simulink model "VectorCtrl_Asynchronous"  (Simulink 7.9)
settings: Solver=ode23tb  StartTime=0.0  StopTime=1  RelTol=1e-3
InitFcn:
  | np=2;
  | fN=50;
  | VN=400;
  | PN=3.7e+04;
  | IN=PN/(VN*1.732);
  | 
  | Rs=0.08233;
  | Lls=0.000724;
  | Rr=0.0503;
  | Llr=0.000724;
  | Lm=0.02711;
  | Ls=Lm+Lls;
  | Lr=Lm+Llr;
  | Kleak=1-Lm*Lm/(Ls*Lr);
  | Tr=Lr/Rr;
  | 
  | Ts=20e-6;
  | fbase=50;
  | Vbase=220*sqrt(3);
  | wbase=2*pi*fbase;
libraries: powerlib x11, simulink x7, powerlib_extras x6
settings Model: Creator=H002220  LastModifiedBy=H002220

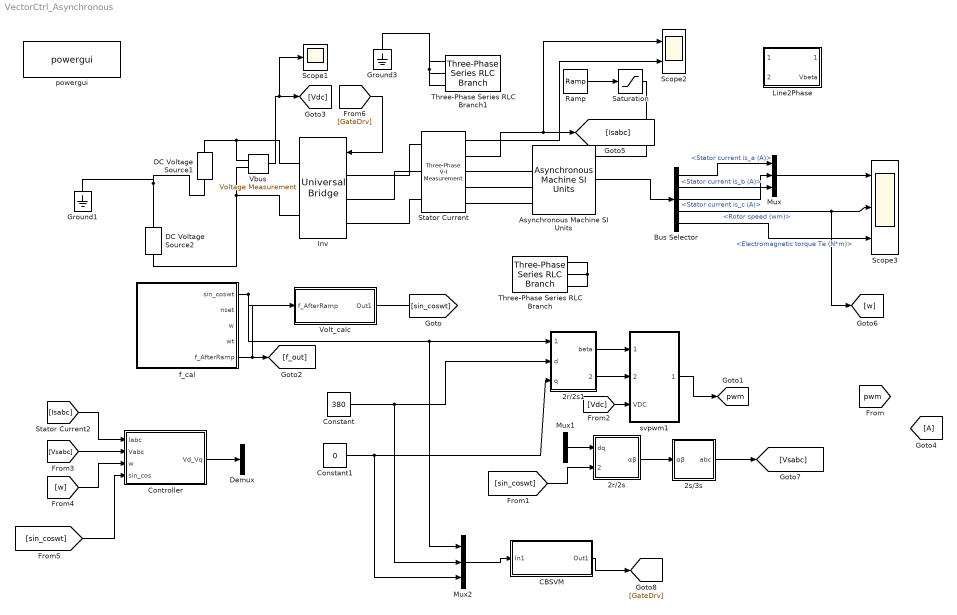
== system VectorCtrl_Asynchronous ==
  2r/2s : Subsystem
  2r/2s1 : Subsystem
  2s/3s : Subsystem
  Asynchronous Machine SI Units : powerlib/Machines/Asynchronous Machine SI Units  PresetModel="18:  50 HP (37KW)   400 V 50Hz 1480 RPM"  MechanicalLoad=Torque Tm  ShowDetailedParameters=on  RotorType=Squirrel-cage  ReferenceFrame=Rotor  NominalParameters=[3.7e+04 400 50]  Stator=[0.08233 0.000724]  Rotor=[0.0503 0.000724]  Cage1=[ 0.022 0.226/377]  Cage2=[ 0.022 0.226/377]  Lm=0.02711  Mechanical=[0.37 0.02791 2]  PolePairs=2  InitialConditions=[1 0 0 0 0 0 0 0]  Units=SI  LoadFlowParameters=1492000  SimulateSaturation=off  Saturation=[14.03593122, 27.81365428, 53.79336849, 72.68890987, 97.98006896, 148.6815601, 215.7428561, 302.9841135, 420.4778367 ; 230, 322, 414, 460, 506, 552, 598, 644, 690]  TsPowergui=0  TsBlock=-1  IterativeModel=Forward Euler  Pmec=0
  Bus Selector : BusSelector  OutputSignals=Stator measurements.Stator current is_a (A),Stator measurements.Stator current is_b (A),Stator measurements.Stator current is_c (A),Mechanical.Rotor speed (wm),Mechanical.Electromagnetic torque Te (N*m)
  CBSVM : Subsystem
  Constant : Constant  Value=380
  Constant1 : Constant  Value=0
  Controller : Subsystem
  DC Voltage Source1 : powerlib/Electrical Sources/DC Voltage Source  Amplitude=300  Measurements=None
  DC Voltage Source2 : powerlib/Electrical Sources/DC Voltage Source  Amplitude=300  Measurements=None
  Demux : Demux  Outputs=2
  Ground1 : powerlib/Elements/Ground  LConnTagsString=a
  Ground3 : powerlib/Elements/Ground  LConnTagsString=a
  Inv : powerlib/Power Electronics/Universal Bridge  Arms=3  SnubberResistance=1e5  SnubberCapacitance=inf  Device=IGBT / Diodes  Ron=1e-3  Lon=0  ForwardVoltages="[  0  0  ]"  ForwardVoltage=0  GTOparameters=[ 10e-6 , 20e-6 ]  IGBTparameters=[ 1e-6 , 2e-6 ]  Measurements=Device voltages  Measurements_2=None  converterType=Rectifier
  Line2Phase : MATLAB Function  TreatAsAtomicUnit=on
  Mux : Mux  Inputs=3
  Mux1 : Mux  Inputs=2
  Mux2 : Mux  Inputs=3
  Ramp : simulink/Sources/Ramp  slope=4  start=0  X0=0
  Saturation : Saturate  UpperLimit=20  LowerLimit=0
  Scope1 : Scope
      settings: SaveName=ScopeData3
  Scope2 : Scope  NumInputPorts=2
      settings: YMin=-5~-5  YMax=5~5  SaveName=ScopeData4
  Scope3 : Scope  NumInputPorts=3
      settings: YMin=-5~-5~-5  YMax=5~5~5  SaveName=ScopeData5
  Stator Current : powerlib/Measurements/Three-Phase V-I Measurement  VoltageMeasurement=phase-to-phase  SetLabelV=off  LabelV=Vabc  Vpu=off  VpuLL=off  CurrentMeasurement=yes  SetLabelI=off  LabelI=Iabc  Ipu=off  Pbase=100e6  Vbase=500e3  OutputType=Complex  PhasorSimulation=off  PSBequivalent=0
  Three-Phase Series RLC Branch : powerlib/Elements/Three-Phase Series RLC Branch  LConnTagsString=A|B|C  RConnTagsString=A|B|C  BranchType=RL  Resistance=1  Inductance=1e-3  Capacitance=1e-6  Measurements=None
  Three-Phase Series RLC Branch1 : powerlib/Elements/Three-Phase Series RLC Branch  LConnTagsString=A|B|C  RConnTagsString=A|B|C  BranchType=R  Resistance=1  Inductance=100*pi*Ls  Capacitance=1e-6  Measurements=None
  Vbus : powerlib/Measurements/Voltage Measurement  PhasorSimulation=off  OutputType=Complex  PSBequivalent=0
  Volt_calc : Subsystem
  f_cal : Subsystem
  powergui : powerlib/powergui  SimulationMode=Discrete  SolverType=Tustin  SampleTime=20e-6  frequency=60  SPID=off  DisableSnubberDevices=off  DisableRonSwitches=off  DisableVfSwitches=off  SwTol=0  Interpol=off  DisplayEquations=off  FunctionMessages=off  frequencyindice=0  Pbase=100e6  ErrMax=1e-4  Iterations=50  UnitsV=kV  UnitsW=MW  echomessages=off  HookPort=off  EnableUseOfTLC=off  x0status=blocks  RestoreLinks=warning  ResistiveCurrentMeasurement=off  Frange=[0:2:500]  Ylog=off  Xlog=on  ShowGrid=off  save=off  variable=ZData  structure=ScopeData4  ZoomFFT=off  StartTime=0.08  cycles=1  DisplayStyle=2  fundamental=50  FreqAxis=on  MaxFrequency=1000  frequencyindicesteady=1  RmsSteady=1  display=off  Ts=0  methode=off
  svpwm1 : Subsystem
  tag scope: pwm=global
  wires:
  2r/2s1/2(alpha) -> svpwm1/2(usaref)
  2r/2s1/1(beta) -> svpwm1/1(usbref)
  [Vdc] -> svpwm1/3(VDC)
  Vbus/1 -> [Vdc], Scope1/1
  Stator Current/2 -> [Isabc], Scope2/1
  f_cal/5(f_AfterRamp) -> [f_out], Volt_calc/1(f_AfterRamp)
  f_cal/1(sin_coswt) -> [sin_coswt], 2r/2s1/1(sin_cos), Mux2/1
  Asynchronous Machine SI Units/1 -> Bus Selector/1
  Ramp/1 -> Saturation/1
  Saturation/1 -> Asynchronous Machine SI Units/1
  Bus Selector/1 -> Mux/1  "<Stator current is_a (A)>"
  Bus Selector/2 -> Mux/2  "<Stator current is_b (A)>"
  Bus Selector/3 -> Mux/3  "<Stator current is_c (A)>"
  Mux/1 -> Scope3/1
  Bus Selector/4 -> Scope3/2, [w]  "<Rotor speed (wm)>"
  Bus Selector/5 -> Scope3/3  "<Electromagnetic torque Te (N*m)>"
  [Isabc] -> Controller/1(Iabc)
  [Vsabc] -> Controller/2(Vabc)
  [w] -> Controller/3(w)
  Mux1/1 -> 2r/2s/1(dq)
  [sin_coswt] -> 2r/2s/2(sin_cos)
  2r/2s/1(αβ) -> 2s/3s/1(αβ)
  2s/3s/1(abc) -> [Vsabc]
  [sin_coswt] -> Controller/4(sin_cos)
  Controller/1(Vd_Vq) -> Demux/1
  Constant/1 -> 2r/2s1/2(d), Mux2/2
  Constant1/1 -> 2r/2s1/3(q), Mux2/3
  Mux2/1 -> CBSVM/1(In1)
  Stator Current/1 -> Scope2/2
  svpwm1/1(6pulse) -> [pwm]
  CBSVM/1(Out1) -> [GateDrv]
  [GateDrv] -> Inv/1
  connections:
  Inv/LConn1 -- Stator Current/LConn1
  Inv/LConn2 -- Stator Current/LConn2
  Inv/LConn3 -- Stator Current/LConn3
  Inv/RConn2 -- Vbus/LConn2 -- DC Voltage Source2/LConn1
  DC Voltage Source1/RConn1 -- Inv/RConn1 -- Vbus/LConn1
  Ground3/LConn1 -- Three-Phase Series RLC Branch1/LConn1 -- Three-Phase Series RLC Branch1/LConn3 -- Three-Phase Series RLC Branch1/LConn2
  DC Voltage Source2/RConn1 -- DC Voltage Source1/LConn1 -- Ground1/LConn1
  Three-Phase Series RLC Branch/RConn1 -- Three-Phase Series RLC Branch/RConn3 -- Three-Phase Series RLC Branch/RConn2
  Stator Current/RConn1 -- Asynchronous Machine SI Units/LConn1
  Stator Current/RConn2 -- Asynchronous Machine SI Units/LConn2
  Stator Current/RConn3 -- Asynchronous Machine SI Units/LConn3

== system VectorCtrl_Asynchronous/2r/2s ==
  dq : Inport
  sin_cos : Inport  Port=2
  Demux : Demux  Outputs=2
  Demux1 : Demux  Outputs=2
  MATLAB Function : MATLAB Function  TreatAsAtomicUnit=on
  Mux : Mux  Inputs=2
  αβ : Outport
  wires:
  Mux/1 -> αβ/1
  Demux/2 -> MATLAB Function/4(coswt)
  Demux/1 -> MATLAB Function/3(sinwt)
  sin_cos/1 -> Demux/1
  dq/1 -> Demux1/1
  Demux1/1 -> MATLAB Function/1(Vd)
  Demux1/2 -> MATLAB Function/2(Vq)
  MATLAB Function/1(Valpha) -> Mux/1
  MATLAB Function/2(Vbeta) -> Mux/2

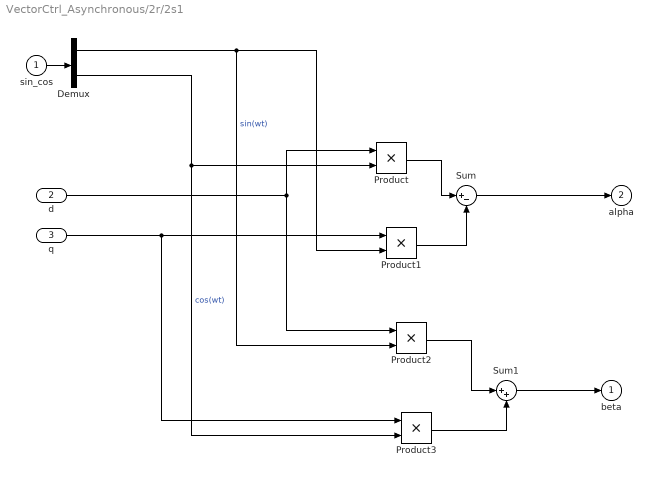
== system VectorCtrl_Asynchronous/2r/2s1 ==
  sin_cos : Inport  PortDimensions=2
  d : Inport  Port=2
  q : Inport  Port=3
  Demux : Demux  Outputs=2
  Product{,1..3} (4 alike) : Product  RndMeth=Zero
  Sum : Sum  Inputs=|+-
  Sum1 : Sum  Inputs=|++
  beta : Outport  InitialOutput=0
  alpha : Outport  Port=2  InitialOutput=0
  wires:
  Sum/1 -> alpha/1
  Demux/1 -> Product1/2, Product2/2  "sin(wt)"
  Demux/2 -> Product/2, Product3/2  "cos(wt)"
  sin_cos/1 -> Demux/1
  d/1 -> Product/1, Product2/1
  q/1 -> Product1/1, Product3/1
  Product/1 -> Sum/1
  Product1/1 -> Sum/2
  Product2/1 -> Sum1/1
  Product3/1 -> Sum1/2
  Sum1/1 -> beta/1

== system VectorCtrl_Asynchronous/2s/3s ==
  αβ : Inport
  Demux : Demux  Outputs=2
  MATLAB Function : MATLAB Function  TreatAsAtomicUnit=on
  Mux : Mux  Inputs=3
  abc : Outport
  wires:
  Demux/1 -> MATLAB Function/1(Valpha)
  Demux/2 -> MATLAB Function/2(Vbeta)
  MATLAB Function/1(Va) -> Mux/1
  MATLAB Function/2(Vb) -> Mux/2
  MATLAB Function/3(Vc) -> Mux/3
  Mux/1 -> abc/1
  αβ/1 -> Demux/1

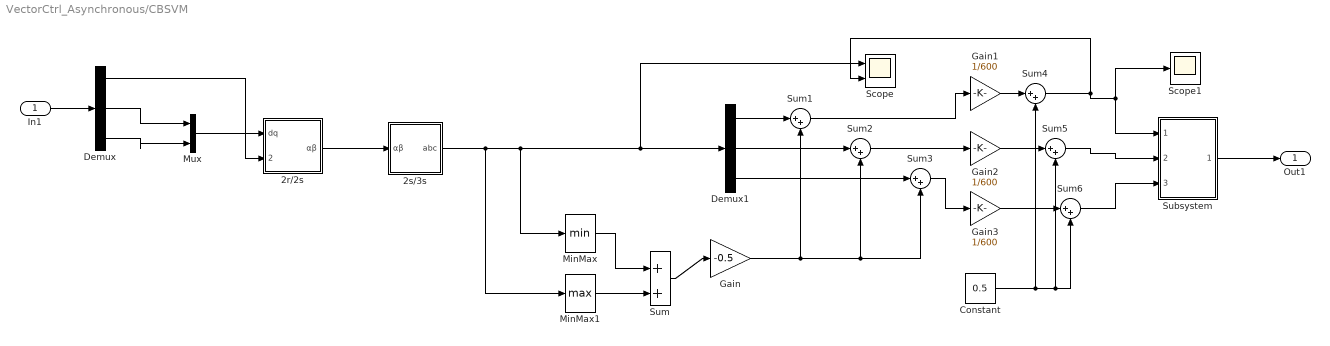
== system VectorCtrl_Asynchronous/CBSVM ==
  In1 : Inport
  2r/2s : Subsystem
  2s/3s : Subsystem
  Constant : Constant  Value=0.5
  Demux : Demux  Outputs=3
  Demux1 : Demux  Outputs=3
  Gain : Gain  Gain=-0.5
  Gain1 : Gain  Gain=1/600
  Gain2 : Gain  Gain=1/600
  Gain3 : Gain  Gain=1/600
  MinMax : MinMax
  MinMax1 : MinMax  Function=max
  Mux : Mux  Inputs=2
  Scope : Scope  NumInputPorts=2
      settings: YMin=-5~-5  YMax=5~5  SaveName=ScopeData12
  Scope1 : Scope
      settings: SaveName=ScopeData14
  Subsystem : Subsystem
  Sum{,1..6} (7 alike) : Sum  Inputs=|++
  Out1 : Outport
  wires:
  In1/1 -> Demux/1
  Demux/2 -> Mux/1
  Demux/3 -> Mux/2
  Mux/1 -> 2r/2s/1(dq)
  Demux/1 -> 2r/2s/2(sin_cos)
  2r/2s/1(αβ) -> 2s/3s/1(αβ)
  2s/3s/1(abc) -> MinMax/1, Demux1/1, Scope/1, MinMax1/1
  MinMax/1 -> Sum/1
  MinMax1/1 -> Sum/2
  Sum/1 -> Gain/1
  Demux1/1 -> Sum1/1
  Demux1/2 -> Sum2/1
  Demux1/3 -> Sum3/1
  Gain/1 -> Sum3/2, Sum2/2, Sum1/2
  Subsystem/1(Out1) -> Out1/1
  Sum1/1 -> Gain1/1
  Sum2/1 -> Gain2/1
  Sum3/1 -> Gain3/1
  Sum4/1 -> Subsystem/1(TCM1), Scope1/1, Scope/2
  Sum5/1 -> Subsystem/2(TCM2)
  Sum6/1 -> Subsystem/3(TCM3)
  Gain1/1 -> Sum4/1
  Gain2/1 -> Sum5/1
  Gain3/1 -> Sum6/1
  Constant/1 -> Sum6/2, Sum5/2, Sum4/2

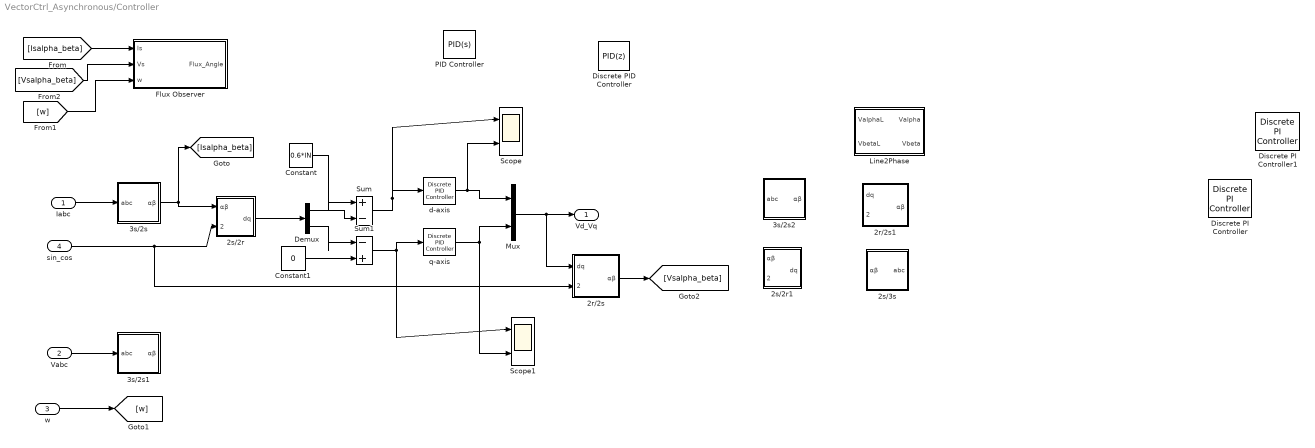
== system VectorCtrl_Asynchronous/Controller ==
  Iabc : Inport
  Vabc : Inport  Port=2
  w : Inport  Port=3
  sin_cos : Inport  Port=4
  2r/2s : Subsystem
  2r/2s1 : Subsystem
  2s/2r : Subsystem
  2s/2r1 : Subsystem
  2s/3s : Subsystem
  3s/2s : Subsystem
  3s/2s1 : Subsystem
  3s/2s2 : Subsystem
  Constant : Constant  Value=0.6*IN
  Constant1 : Constant  Value=0
  Demux : Demux  Outputs=2
  Discrete PI Controller : powerlib_extras/Discrete  Control Blocks/Discrete PI Controller  Kp=0.1  Ki=1  Par_Limits=[1e6 -1e6]  Init=0  Ts=50e-6
  Discrete PI Controller1 : powerlib_extras/Discrete  Control Blocks/Discrete PI Controller  Kp=0.1  Ki=1  Par_Limits=[1e6 -1e6]  Init=0  Ts=50e-6
  Discrete PID Controller : simulink/Continuous/PID Controller  Controller=PID  TimeDomain=Discrete-time  SampleTime=1  IntegratorMethod=Forward Euler  FilterMethod=Forward Euler  Form=Parallel  P=1  I=1  D=0  N=100  InitialConditionSource=internal  InitialConditionForIntegrator=0  InitialConditionForFilter=0  ExternalReset=none  LimitOutput=off  UpperSaturationLimit=inf  LowerSaturationLimit=-inf  LinearizeAsGain=off  AntiWindupMode=none  Kb=1  TrackingMode=off  Kt=1  PParamMin=[]  PParamMax=[]  IParamMin=[]  IParamMax=[]  DParamMin=[]  DParamMax=[]  NParamMin=[]  NParamMax=[]  KbParamMin=[]  KbParamMax=[]  KtParamMin=[]  KtParamMax=[]  POutMin=[]  POutMax=[]  IOutMin=[]  IOutMax=[]  DOutMin=[]  DOutMax=[]  NOutMin=[]  NOutMax=[]  KbOutMin=[]  KbOutMax=[]  KtOutMin=[]  KtOutMax=[]  IntegratorOutMin=[]  IntegratorOutMax=[]  FilterOutMin=[]  FilterOutMax=[]  SumOutMin=[]  SumOutMax=[]  SumI1OutMin=[]  SumI1OutMax=[]  SumI2OutMin=[]  SumI2OutMax=[]  SumI3OutMin=[]  SumI3OutMax=[]  SumDOutMin=[]  SumDOutMax=[]  SaturationOutMin=[]  SaturationOutMax=[]  IntegratorContinuousStateAttributes=''  IntegratorStateMustResolveToSignalObject=off  IntegratorRTWStateStorageClass=Auto  FilterContinuousStateAttributes=''  FilterStateMustResolveToSignalObject=off  FilterRTWStateStorageClass=Auto
  Flux Observer : Subsystem
  Line2Phase : MATLAB Function  TreatAsAtomicUnit=on
  Mux : Mux  Inputs=2
  PID Controller : simulink/Continuous/PID Controller  Controller=PID  TimeDomain=Continuous-time  SampleTime=1  IntegratorMethod=Forward Euler  FilterMethod=Forward Euler  Form=Parallel  P=1  I=1  D=0  N=100  InitialConditionSource=internal  InitialConditionForIntegrator=0  InitialConditionForFilter=0  ExternalReset=none  LimitOutput=off  UpperSaturationLimit=inf  LowerSaturationLimit=-inf  LinearizeAsGain=off  AntiWindupMode=none  Kb=1  TrackingMode=off  Kt=1  PParamMin=[]  PParamMax=[]  IParamMin=[]  IParamMax=[]  DParamMin=[]  DParamMax=[]  NParamMin=[]  NParamMax=[]  KbParamMin=[]  KbParamMax=[]  KtParamMin=[]  KtParamMax=[]  POutMin=[]  POutMax=[]  IOutMin=[]  IOutMax=[]  DOutMin=[]  DOutMax=[]  NOutMin=[]  NOutMax=[]  KbOutMin=[]  KbOutMax=[]  KtOutMin=[]  KtOutMax=[]  IntegratorOutMin=[]  IntegratorOutMax=[]  FilterOutMin=[]  FilterOutMax=[]  SumOutMin=[]  SumOutMax=[]  SumI1OutMin=[]  SumI1OutMax=[]  SumI2OutMin=[]  SumI2OutMax=[]  SumI3OutMin=[]  SumI3OutMax=[]  SumDOutMin=[]  SumDOutMax=[]  SaturationOutMin=[]  SaturationOutMax=[]  IntegratorContinuousStateAttributes=''  IntegratorStateMustResolveToSignalObject=off  IntegratorRTWStateStorageClass=Auto  FilterContinuousStateAttributes=''  FilterStateMustResolveToSignalObject=off  FilterRTWStateStorageClass=Auto
  Scope : Scope  NumInputPorts=2
      settings: YMin=-5~-5  YMax=5~5  SaveName=ScopeData7
  Scope1 : Scope  NumInputPorts=2
      settings: YMin=-5~-5  YMax=5~5  SaveName=ScopeData11
  Sum : Sum  Inputs=|+-
  Sum1 : Sum  Inputs=|-+
  d-axis : powerlib_extras/Discrete  Control Blocks/Discrete PID Controller  Kp=100  Ki=2  Kd=0  TcD=Ts/2  Par_Limits=[600 -600]  Init=0  Ts=Ts/2
  q-axis : powerlib_extras/Discrete  Control Blocks/Discrete PID Controller  Kp=100  Ki=2  Kd=0  TcD=Ts/2  Par_Limits=[600 -600]  Init=0  Ts=Ts/2
  Vd_Vq : Outport
  wires:
  Iabc/1 -> 3s/2s/1(abc)
  3s/2s/1(αβ) -> [Isalpha_beta], 2s/2r/1(αβ)
  [Isalpha_beta] -> Flux Observer/1(Is)
  w/1 -> [w]
  [w] -> Flux Observer/3(w)
  Vabc/1 -> 3s/2s1/1(abc)
  [Vsalpha_beta] -> Flux Observer/2(Vs)
  sin_cos/1 -> 2s/2r/2(sin_cos), 2r/2s/2(sin_cos)
  2s/2r/1(dq) -> Demux/1
  Demux/1 -> Sum/2
  Demux/2 -> Sum1/1
  Constant/1 -> Sum/1
  Constant1/1 -> Sum1/2
  Sum1/1 -> q-axis/1, Scope1/1
  Sum/1 -> d-axis/1, Scope/1
  d-axis/1 -> Mux/1, Scope/2
  q-axis/1 -> Mux/2, Scope1/2
  Mux/1 -> Vd_Vq/1, 2r/2s/1(dq)
  2r/2s/1(αβ) -> [Vsalpha_beta]

== system VectorCtrl_Asynchronous/Volt_calc ==
  f_AfterRamp : Inport
  Constant : Constant  Value=0.1*fbase
  Gain : Gain  Gain=1/fbase
  Gain1 : Gain  Gain=Vbase
  Ramp : simulink/Sources/Ramp  slope=1  start=0  X0=0
  Scope : Scope
      settings: SaveName=ScopeData6
  Switch : Switch
  Out1 : Outport
  wires:
  Gain/1 -> Gain1/1
  Gain1/1 -> Out1/1, Scope/1
  Ramp/1 -> Switch/2
  f_AfterRamp/1 -> Switch/1
  Constant/1 -> Switch/3
  Switch/1 -> Gain/1

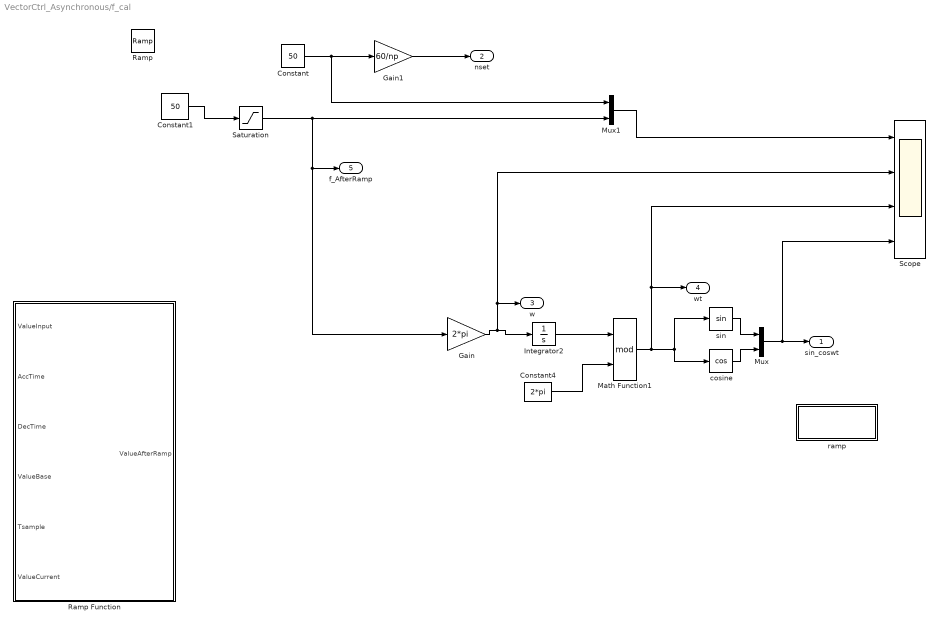
== system VectorCtrl_Asynchronous/f_cal ==
  Constant : Constant  Value=50
  Constant1 : Constant  Value=50
  Constant4 : Constant  Value=2*pi
  Gain : Gain  Gain=2*pi
  Gain1 : Gain  Gain=60/np
  Integrator2 : Integrator
  Math Function1 : Math  Operator=mod  SaturateOnIntegerOverflow=on
  Mux : Mux  Inputs=2
  Mux1 : Mux  Inputs=2
  Ramp : simulink/Sources/Ramp  slope=10  start=0  X0=0
  Ramp Function : MATLAB Function  TreatAsAtomicUnit=on
  Saturation : Saturate  UpperLimit=50  LowerLimit=0
  Scope : Scope  NumInputPorts=4
      settings: YMin=-5~-5~-5~-5  YMax=5~5~5~5
  cosine : Trigonometry  Operator=cos
  ramp : Subsystem
  sin : Trigonometry
  sin_coswt : Outport
  nset : Outport  Port=2
  w : Outport  Port=3
  wt : Outport  Port=4
  f_AfterRamp : Outport  Port=5
  wires:
  sin/1 -> Mux/1
  cosine/1 -> Mux/2
  Mux/1 -> sin_coswt/1, Scope/4
  Gain1/1 -> nset/1
  Mux1/1 -> Scope/1
  Constant4/1 -> Math Function1/2
  Integrator2/1 -> Math Function1/1
  Gain/1 -> Integrator2/1, w/1, Scope/2
  Math Function1/1 -> sin/1, cosine/1, wt/1, Scope/3
  Constant/1 -> Gain1/1, Mux1/1
  Saturation/1 -> Mux1/2, f_AfterRamp/1, Gain/1
  Constant1/1 -> Saturation/1

== system VectorCtrl_Asynchronous/svpwm1 ==
  usbref : Inport
  usaref : Inport  Port=2
  VDC : Inport  Port=3
  Campare Time Calculate : Subsystem
  Memory : Memory
  On/Off Delay : powerlib_extras/Control  Blocks/On//Off Delay  type_delay=On delay  delay=1e-6  ic=0
  Sector Calculate : Subsystem
  Subsystem : Subsystem
  T : Constant  Value=1/5000
  T1,T2 Calculate : Subsystem
  x,y,z Calculate : Subsystem
  6pulse : Outport
  wires:
  usbref/1 -> Sector Calculate/1(usbref), x,y,z Calculate/1(usbref)
  usaref/1 -> Sector Calculate/2(usaref), x,y,z Calculate/2(usaref)
  Sector Calculate/1(N) -> T1,T2 Calculate/1(N), Campare Time Calculate/1(N)
  x,y,z Calculate/1(x) -> T1,T2 Calculate/2(x)
  x,y,z Calculate/2(y) -> T1,T2 Calculate/3(y)
  x,y,z Calculate/3(z) -> T1,T2 Calculate/4(z)
  T1,T2 Calculate/1(T1) -> Campare Time Calculate/2(T1)
  T1,T2 Calculate/2(T2) -> Campare Time Calculate/3(T2)
  Campare Time Calculate/1(TCM1) -> Subsystem/1(TCM1)
  Campare Time Calculate/2(TCM2) -> Subsystem/2(TCM2)
  Campare Time Calculate/3(TCM3) -> Subsystem/3(TCM3)
  Subsystem/1(Out1) -> Memory/1
  T/1 -> x,y,z Calculate/3(T), T1,T2 Calculate/5(T), Campare Time Calculate/4(T)
  VDC/1 -> x,y,z Calculate/4(VDC)
  Memory/1 -> On/Off Delay/1
  On/Off Delay/1 -> 6pulse/1

== system VectorCtrl_Asynchronous/CBSVM/2r/2s ==
  dq : Inport
  sin_cos : Inport  Port=2
  Demux : Demux  Outputs=2
  Demux1 : Demux  Outputs=2
  MATLAB Function : MATLAB Function  TreatAsAtomicUnit=on
  Mux : Mux  Inputs=2
  αβ : Outport
  wires:
  Mux/1 -> αβ/1
  Demux/2 -> MATLAB Function/4(coswt)
  Demux/1 -> MATLAB Function/3(sinwt)
  sin_cos/1 -> Demux/1
  dq/1 -> Demux1/1
  Demux1/1 -> MATLAB Function/1(Vd)
  Demux1/2 -> MATLAB Function/2(Vq)
  MATLAB Function/1(Valpha) -> Mux/1
  MATLAB Function/2(Vbeta) -> Mux/2

== system VectorCtrl_Asynchronous/CBSVM/2s/3s ==
  αβ : Inport
  Demux : Demux  Outputs=2
  MATLAB Function : MATLAB Function  TreatAsAtomicUnit=on
  Mux : Mux  Inputs=3
  abc : Outport
  wires:
  Demux/1 -> MATLAB Function/1(Valpha)
  Demux/2 -> MATLAB Function/2(Vbeta)
  MATLAB Function/1(Va) -> Mux/1
  MATLAB Function/2(Vb) -> Mux/2
  MATLAB Function/3(Vc) -> Mux/3
  Mux/1 -> abc/1
  αβ/1 -> Demux/1

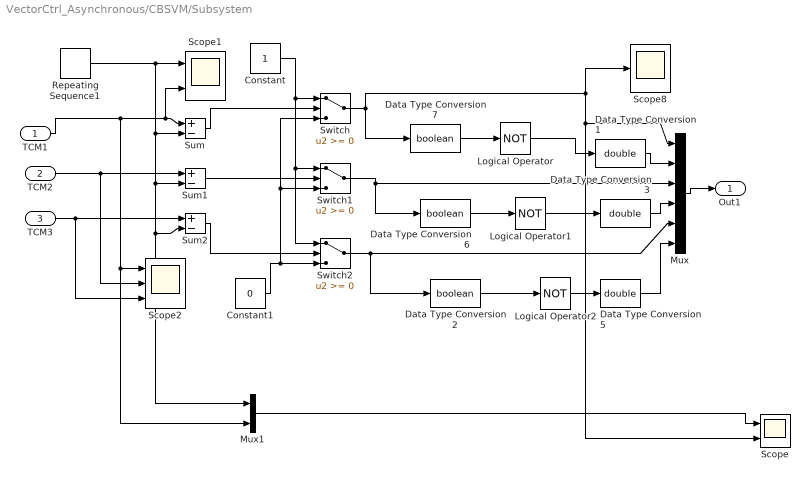
== system VectorCtrl_Asynchronous/CBSVM/Subsystem ==
  TCM1 : Inport
  TCM2 : Inport  Port=2
  TCM3 : Inport  Port=3
  Constant : Constant
  Constant1 : Constant  Value=0
  Data Type Conversion1 : DataTypeConversion  OutDataTypeStr=double  SaturateOnIntegerOverflow=on  RndMeth=Zero
  Data Type Conversion2 : DataTypeConversion  OutDataTypeStr=boolean  SaturateOnIntegerOverflow=on  RndMeth=Zero
  Data Type Conversion3 : DataTypeConversion  OutDataTypeStr=double  SaturateOnIntegerOverflow=on  RndMeth=Zero
  Data Type Conversion5 : DataTypeConversion  OutDataTypeStr=double  SaturateOnIntegerOverflow=on  RndMeth=Zero
  Data Type Conversion6 : DataTypeConversion  OutDataTypeStr=boolean  SaturateOnIntegerOverflow=on  RndMeth=Zero
  Data Type Conversion7 : DataTypeConversion  OutDataTypeStr=boolean  SaturateOnIntegerOverflow=on  RndMeth=Zero
  Logical Operator : Logic  Operator=NOT  AllPortsSameDT=off
  Logical Operator1 : Logic  Operator=NOT  AllPortsSameDT=off
  Logical Operator2 : Logic  Operator=NOT  AllPortsSameDT=off
  Mux : Mux  Inputs=6
  Mux1 : Mux  Inputs=2
  Repeating Sequence1 : simulink/Sources/Repeating Sequence  rep_seq_t=[0 1/10000 1/5000]  rep_seq_y=[0 1 0]
  Scope : Scope  NumInputPorts=2
      settings: YMin=-5~-5  YMax=5~5  SaveName=ScopeData21
  Scope1 : Scope  NumInputPorts=2
      settings: TimeRange=0.028  YMin=0~2.45e-005  YMax=1.2~2.64e-005  SaveName=ScopeData15
  Scope2 : Scope  NumInputPorts=3
      settings: TimeRange=1  YMin=2.25e-005~2.25e-005~2.25e-05  YMax=6e-005~6e-005~6e-05  SaveName=ScopeData19
  Scope8 : Scope
      settings: TimeRange=0.07000000000000001  YMin=0  YMax=2  SaveName=ScopeData13
  Sum : Sum  Inputs=+-  SaturateOnIntegerOverflow=on
  Sum1 : Sum  Inputs=+-  SaturateOnIntegerOverflow=on
  Sum2 : Sum  Inputs=+-  SaturateOnIntegerOverflow=on
  Switch : Switch  SaturateOnIntegerOverflow=on
  Switch1 : Switch  SaturateOnIntegerOverflow=on
  Switch2 : Switch  SaturateOnIntegerOverflow=on
  Out1 : Outport
  wires:
  Constant/1 -> Switch/1, Switch1/1, Switch2/1
  Constant1/1 -> Switch2/3, Switch/3, Switch1/3
  Repeating Sequence1/1 -> Scope1/1, Sum/2, Sum1/2, Sum2/2, Mux1/1
  TCM1/1 -> Sum/1, Scope1/2, Scope2/1, Mux1/2
  TCM2/1 -> Sum1/1, Scope2/2
  TCM3/1 -> Sum2/1, Scope2/3
  Sum/1 -> Switch/2
  Sum1/1 -> Switch1/2
  Sum2/1 -> Switch2/2
  Mux/1 -> Out1/1
  Switch/1 -> Scope8/1, Mux/1, Scope/2, Data Type Conversion7/1
  Switch1/1 -> Mux/3, Data Type Conversion6/1
  Switch2/1 -> Data Type Conversion2/1, Mux/5
  Logical Operator2/1 -> Data Type Conversion5/1
  Logical Operator1/1 -> Data Type Conversion3/1
  Logical Operator/1 -> Data Type Conversion1/1
  Data Type Conversion1/1 -> Mux/2
  Data Type Conversion3/1 -> Mux/4
  Data Type Conversion5/1 -> Mux/6
  Data Type Conversion7/1 -> Logical Operator/1
  Data Type Conversion6/1 -> Logical Operator1/1
  Data Type Conversion2/1 -> Logical Operator2/1
  Mux1/1 -> Scope/1

== system VectorCtrl_Asynchronous/Controller/2r/2s ==
  dq : Inport
  sin_cos : Inport  Port=2
  Demux : Demux  Outputs=2
  Demux1 : Demux  Outputs=2
  MATLAB Function : MATLAB Function  TreatAsAtomicUnit=on
  Mux : Mux  Inputs=2
  αβ : Outport
  wires:
  Mux/1 -> αβ/1
  Demux/2 -> MATLAB Function/4(coswt)
  Demux/1 -> MATLAB Function/3(sinwt)
  sin_cos/1 -> Demux/1
  dq/1 -> Demux1/1
  Demux1/1 -> MATLAB Function/1(Vd)
  Demux1/2 -> MATLAB Function/2(Vq)
  MATLAB Function/1(Valpha) -> Mux/1
  MATLAB Function/2(Vbeta) -> Mux/2

== system VectorCtrl_Asynchronous/Controller/2r/2s1 ==
  dq : Inport
  sin_cos : Inport  Port=2
  Demux : Demux  Outputs=2
  Demux1 : Demux  Outputs=2
  MATLAB Function : MATLAB Function  TreatAsAtomicUnit=on
  Mux : Mux  Inputs=2
  αβ : Outport
  wires:
  MATLAB Function/2(Vbeta) -> Mux/2
  MATLAB Function/1(Valpha) -> Mux/1
  Demux1/2 -> MATLAB Function/2(Vq)
  Demux1/1 -> MATLAB Function/1(Vd)
  dq/1 -> Demux1/1
  sin_cos/1 -> Demux/1
  Demux/1 -> MATLAB Function/3(sinwt)
  Demux/2 -> MATLAB Function/4(coswt)
  Mux/1 -> αβ/1

== system VectorCtrl_Asynchronous/Controller/2s/2r ==
  αβ : Inport
  sin_cos : Inport  Port=2
  Demux : Demux  Outputs=2
  Demux1 : Demux  Outputs=2
  MATLAB Function : MATLAB Function  TreatAsAtomicUnit=on
  Mux : Mux  Inputs=2
  dq : Outport
  wires:
  αβ/1 -> Demux1/1
  sin_cos/1 -> Demux/1
  Demux/1 -> MATLAB Function/3(sinwt)
  Demux/2 -> MATLAB Function/4(coswt)
  MATLAB Function/1(Vd) -> Mux/1
  MATLAB Function/2(Vq) -> Mux/2
  Mux/1 -> dq/1
  Demux1/2 -> MATLAB Function/2(Vbeta)
  Demux1/1 -> MATLAB Function/1(Valpha)

== system VectorCtrl_Asynchronous/Controller/2s/2r1 ==
  αβ : Inport
  sin_cos : Inport  Port=2
  Demux : Demux  Outputs=2
  Demux1 : Demux  Outputs=2
  MATLAB Function : MATLAB Function  TreatAsAtomicUnit=on
  Mux : Mux  Inputs=2
  dq : Outport
  wires:
  Demux1/1 -> MATLAB Function/1(Valpha)
  Demux1/2 -> MATLAB Function/2(Vbeta)
  Mux/1 -> dq/1
  MATLAB Function/2(Vq) -> Mux/2
  MATLAB Function/1(Vd) -> Mux/1
  Demux/2 -> MATLAB Function/4(coswt)
  Demux/1 -> MATLAB Function/3(sinwt)
  sin_cos/1 -> Demux/1
  αβ/1 -> Demux1/1

== system VectorCtrl_Asynchronous/Controller/2s/3s ==
  αβ : Inport
  Demux : Demux  Outputs=2
  MATLAB Function : MATLAB Function  TreatAsAtomicUnit=on
  Mux : Mux  Inputs=3
  abc : Outport
  wires:
  Demux/1 -> MATLAB Function/1(Valpha)
  Demux/2 -> MATLAB Function/2(Vbeta)
  MATLAB Function/1(Va) -> Mux/1
  MATLAB Function/2(Vb) -> Mux/2
  MATLAB Function/3(Vc) -> Mux/3
  Mux/1 -> abc/1
  αβ/1 -> Demux/1

== system VectorCtrl_Asynchronous/Controller/3s/2s ==
  abc : Inport
  Demux : Demux  Outputs=3
  MATLAB Function : MATLAB Function  TreatAsAtomicUnit=on
  Mux : Mux  Inputs=2
  αβ : Outport
  wires:
  abc/1 -> Demux/1
  Mux/1 -> αβ/1
  Demux/1 -> MATLAB Function/1(Va)
  Demux/2 -> MATLAB Function/2(Vb)
  Demux/3 -> MATLAB Function/3(Vc)
  MATLAB Function/1(Valpha) -> Mux/1
  MATLAB Function/2(Vbeta) -> Mux/2

== system VectorCtrl_Asynchronous/Controller/3s/2s1 ==
  abc : Inport
  Demux : Demux  Outputs=3
  MATLAB Function : MATLAB Function  TreatAsAtomicUnit=on
  Mux : Mux  Inputs=2
  αβ : Outport
  wires:
  MATLAB Function/2(Vbeta) -> Mux/2
  MATLAB Function/1(Valpha) -> Mux/1
  Demux/3 -> MATLAB Function/3(Vc)
  Demux/2 -> MATLAB Function/2(Vb)
  Demux/1 -> MATLAB Function/1(Va)
  Mux/1 -> αβ/1
  abc/1 -> Demux/1

== system VectorCtrl_Asynchronous/Controller/3s/2s2 ==
  abc : Inport
  Demux : Demux  Outputs=3
  MATLAB Function : MATLAB Function  TreatAsAtomicUnit=on
  Mux : Mux  Inputs=2
  αβ : Outport
  wires:
  abc/1 -> Demux/1
  Mux/1 -> αβ/1
  Demux/1 -> MATLAB Function/1(Va)
  Demux/2 -> MATLAB Function/2(Vb)
  Demux/3 -> MATLAB Function/3(Vc)
  MATLAB Function/1(Valpha) -> Mux/1
  MATLAB Function/2(Vbeta) -> Mux/2

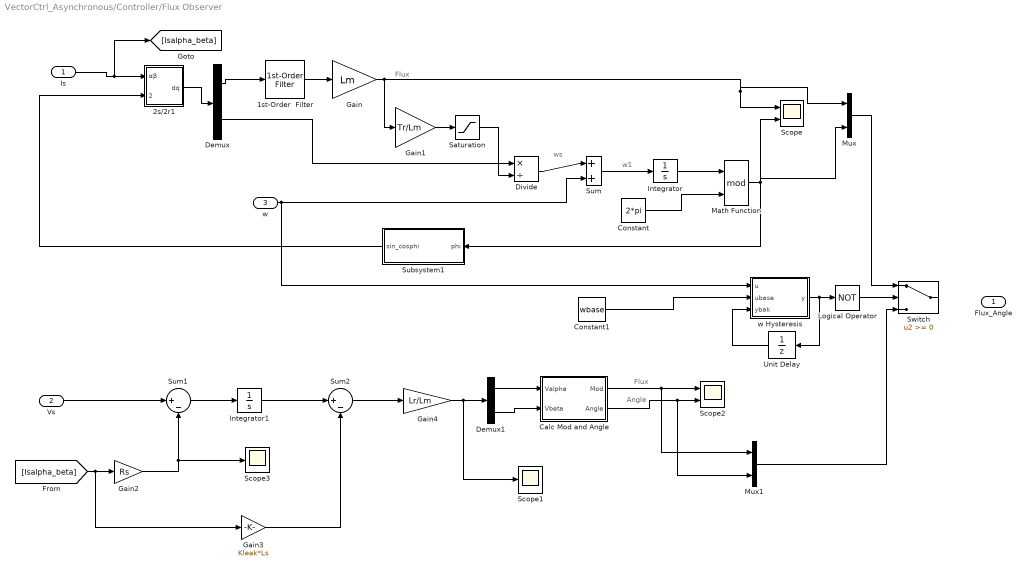
== system VectorCtrl_Asynchronous/Controller/Flux Observer ==
  note: Flux
  note: ws
  note: w1
  note: Flux
  note: Angle
  Is : Inport
  Vs : Inport  Port=2
  w : Inport  Port=3
  1st-Order  Filter : powerlib_extras/Control  Blocks/1st-Order  Filter  FilterType=Lowpass  Tc=Tr  Initialize=off  Vac_Init=[0.8 -25 60]  Vdc_Init=-0.4  PlotResponse=off  param1=[1 500 1]
  2s/2r1 : Subsystem
  Calc Mod and Angle : MATLAB Function  TreatAsAtomicUnit=on
  Constant : Constant  Value=2*pi
  Constant1 : Constant  Value=wbase
  Demux : Demux  Outputs=2
  Demux1 : Demux  Outputs=2
  Divide : Product  Inputs=*/
  Gain : Gain  Gain=Lm
  Gain1 : Gain  Gain=Tr/Lm
  Gain2 : Gain  Gain=Rs
  Gain3 : Gain  Gain=Kleak*Ls
  Gain4 : Gain  Gain=Lr/Lm
  Integrator : Integrator  InitialCondition=0.1
  Integrator1 : Integrator
  Logical Operator : Logic  Operator=NOT  AllPortsSameDT=off  OutDataTypeStr=boolean
  Math Function : Math  Operator=mod  SaturateOnIntegerOverflow=on
  Mux : Mux  Inputs=2
  Mux1 : Mux  Inputs=2
  Saturation : Saturate  UpperLimit=1e3  LowerLimit=0.0001
  Scope : Scope  NumInputPorts=2
      settings: YMin=-5~-5  YMax=5~5  SaveName=ScopeData2
  Scope1 : Scope
      settings: SaveName=ScopeData8
  Scope2 : Scope  NumInputPorts=2
      settings: YMin=-5~-5  YMax=5~5  SaveName=ScopeData9
  Scope3 : Scope
      settings: SaveName=ScopeData10
  Subsystem1 : Subsystem
  Sum : Sum  Inputs=|++
  Sum1 : Sum  Inputs=|+-
  Sum2 : Sum  Inputs=|+-
  Switch : Switch
  Unit Delay : UnitDelay  SampleTime=-1
  w Hysteresis : MATLAB Function  TreatAsAtomicUnit=on
  Flux_Angle : Outport
  wires:
  Is/1 -> 2s/2r1/1(αβ), [Isalpha_beta]
  2s/2r1/1(dq) -> Demux/1
  Demux/1 -> 1st-Order  Filter/1
  1st-Order  Filter/1 -> Gain/1
  Gain/1 -> Gain1/1, Scope/1, Mux/1
  Demux/2 -> Divide/1
  Subsystem1/1(sin_cosphi) -> 2s/2r1/2(sin_cos)
  Divide/1 -> Sum/1
  w/1 -> Sum/2, w Hysteresis/1(u)
  Sum/1 -> Integrator/1
  Gain1/1 -> Saturation/1
  Integrator/1 -> Math Function/1
  Constant/1 -> Math Function/2
  Math Function/1 -> Scope/2, Subsystem1/1(phi), Mux/2
  [Isalpha_beta] -> Gain2/1, Gain3/1
  Vs/1 -> Sum1/1
  Gain2/1 -> Sum1/2, Scope3/1
  Sum1/1 -> Integrator1/1
  Integrator1/1 -> Sum2/1
  Gain3/1 -> Sum2/2
  Sum2/1 -> Gain4/1
  Gain4/1 -> Scope1/1, Demux1/1
  Demux1/1 -> Calc Mod and Angle/1(Valpha)
  Demux1/2 -> Calc Mod and Angle/2(Vbeta)
  Calc Mod and Angle/1(Mod) -> Scope2/1, Mux1/1
  Calc Mod and Angle/2(Angle) -> Scope2/2, Mux1/2
  Constant1/1 -> w Hysteresis/2(ubase)
  Unit Delay/1 -> w Hysteresis/3(ybak)
  w Hysteresis/1(y) -> Logical Operator/1, Unit Delay/1
  Logical Operator/1 -> Switch/2
  Mux1/1 -> Switch/3
  Mux/1 -> Switch/1
  Saturation/1 -> Divide/2

== system VectorCtrl_Asynchronous/f_cal/ramp ==
  Constant : Constant  Value=fbase
  Constant1 : Constant  Value=Ts
  Constant2 : Constant
  Constant3 : Constant
  Constant4 : Constant  Value=50
  MATLAB Function : MATLAB Function  TreatAsAtomicUnit=on
  Scope : Scope
  Unit Delay : UnitDelay  SampleTime=-1
  wires:
  Constant1/1 -> MATLAB Function/5(Tsample)
  Constant/1 -> MATLAB Function/4(ValueBase)
  Constant2/1 -> MATLAB Function/3(DecTime)
  Constant3/1 -> MATLAB Function/2(AccTime)
  Constant4/1 -> MATLAB Function/1(ValueInput)
  MATLAB Function/1(ValueAfterRamp) -> Scope/1, Unit Delay/1
  Unit Delay/1 -> MATLAB Function/6(ValueCurrent)

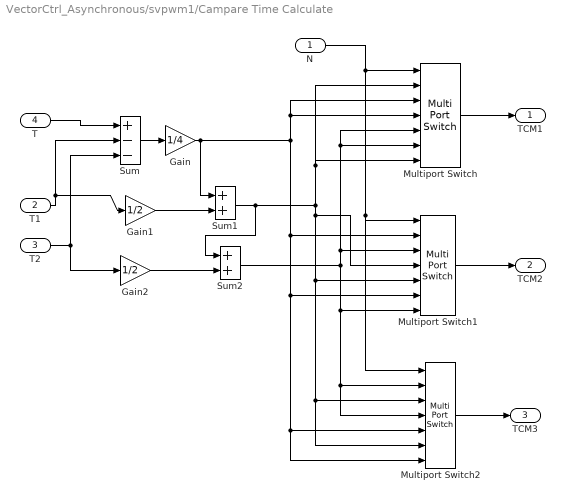
== system VectorCtrl_Asynchronous/svpwm1/Campare Time Calculate ==
  N : Inport
  T1 : Inport  Port=2
  T2 : Inport  Port=3
  T : Inport  Port=4
  Gain : Gain  Gain=1/4  SaturateOnIntegerOverflow=on  OutDataTypeStr=Inherit: Same as input  ParamDataTypeStr=Inherit: Same as input
  Gain1 : Gain  Gain=1/2  SaturateOnIntegerOverflow=on  OutDataTypeStr=Inherit: Same as input  ParamDataTypeStr=Inherit: Same as input
  Gain2 : Gain  Gain=1/2  SaturateOnIntegerOverflow=on  OutDataTypeStr=Inherit: Same as input  ParamDataTypeStr=Inherit: Same as input
  Multiport Switch : MultiPortSwitch  Inputs=6  zeroidx=off  SaturateOnIntegerOverflow=on
  Multiport Switch1 : MultiPortSwitch  Inputs=6  zeroidx=off  SaturateOnIntegerOverflow=on
  Multiport Switch2 : MultiPortSwitch  Inputs=6  zeroidx=off  SaturateOnIntegerOverflow=on
  Sum : Sum  Inputs=+--  SaturateOnIntegerOverflow=on
  Sum1 : Sum  SaturateOnIntegerOverflow=on
  Sum2 : Sum  SaturateOnIntegerOverflow=on
  TCM1 : Outport
  TCM2 : Outport  Port=2
  TCM3 : Outport  Port=3
  wires:
  T/1 -> Sum/1
  T1/1 -> Sum/2, Gain1/1
  T2/1 -> Sum/3, Gain2/1
  Sum/1 -> Gain/1
  Gain/1 -> Sum1/1, Multiport Switch1/2, Multiport Switch2/5, Multiport Switch2/7, Multiport Switch1/6, Multiport Switch/3, Multiport Switch/4
  Gain1/1 -> Sum1/2
  Gain2/1 -> Sum2/2
  Multiport Switch1/1 -> TCM2/1
  Multiport Switch/1 -> TCM1/1
  Multiport Switch2/1 -> TCM3/1
  N/1 -> Multiport Switch/1, Multiport Switch2/1, Multiport Switch1/1
  Sum1/1 -> Sum2/1, Multiport Switch1/4, Multiport Switch2/3, Multiport Switch2/6, Multiport Switch1/5, Multiport Switch/2, Multiport Switch/7
  Sum2/1 -> Multiport Switch1/3, Multiport Switch/6, Multiport Switch/5, Multiport Switch2/2, Multiport Switch2/4, Multiport Switch1/7

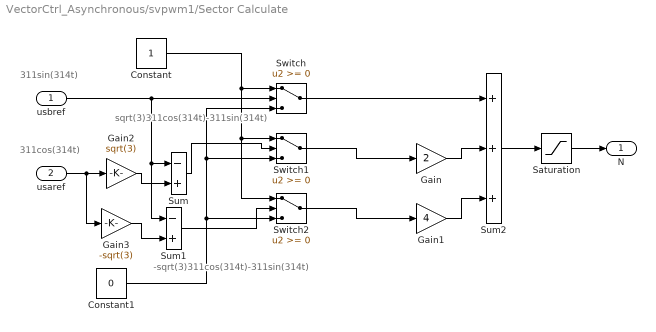
== system VectorCtrl_Asynchronous/svpwm1/Sector Calculate ==
  note: 311sin(314t)
  note: 311cos(314t)
  note: sqrt(3)311cos(314t)-311sin(314t)
  note: -sqrt(3)311cos(314t)-311sin(314t)
  usbref : Inport
  usaref : Inport  Port=2
  Constant : Constant
  Constant1 : Constant  Value=0
  Gain : Gain  Gain=2  SaturateOnIntegerOverflow=on  OutDataTypeStr=Inherit: Same as input  ParamDataTypeStr=Inherit: Same as input
  Gain1 : Gain  Gain=4  SaturateOnIntegerOverflow=on  OutDataTypeStr=Inherit: Same as input  ParamDataTypeStr=Inherit: Same as input
  Gain2 : Gain  Gain=sqrt(3)  SaturateOnIntegerOverflow=on  OutDataTypeStr=Inherit: Same as input  ParamDataTypeStr=Inherit: Same as input
  Gain3 : Gain  Gain=-sqrt(3)  SaturateOnIntegerOverflow=on  OutDataTypeStr=Inherit: Same as input  ParamDataTypeStr=Inherit: Same as input
  Saturation : Saturate  UpperLimit=6  LowerLimit=1
  Sum : Sum  Inputs=-+  SaturateOnIntegerOverflow=on
  Sum1 : Sum  Inputs=-+  SaturateOnIntegerOverflow=on
  Sum2 : Sum  Inputs=+++  SaturateOnIntegerOverflow=on
  Switch : Switch  SaturateOnIntegerOverflow=on
  Switch1 : Switch  SaturateOnIntegerOverflow=on
  Switch2 : Switch  SaturateOnIntegerOverflow=on
  N : Outport
  wires:
  Constant/1 -> Switch/1, Switch1/1, Switch2/1
  usbref/1 -> Sum/1, Sum1/1, Switch/2
  Constant1/1 -> Switch/3, Switch1/3, Switch2/3
  usaref/1 -> Gain2/1, Gain3/1
  Gain2/1 -> Sum/2
  Gain3/1 -> Sum1/2
  Sum/1 -> Switch1/2
  Sum1/1 -> Switch2/2
  Switch1/1 -> Gain/1
  Switch/1 -> Sum2/1
  Gain/1 -> Sum2/2
  Gain1/1 -> Sum2/3
  Switch2/1 -> Gain1/1
  Sum2/1 -> Saturation/1
  Saturation/1 -> N/1

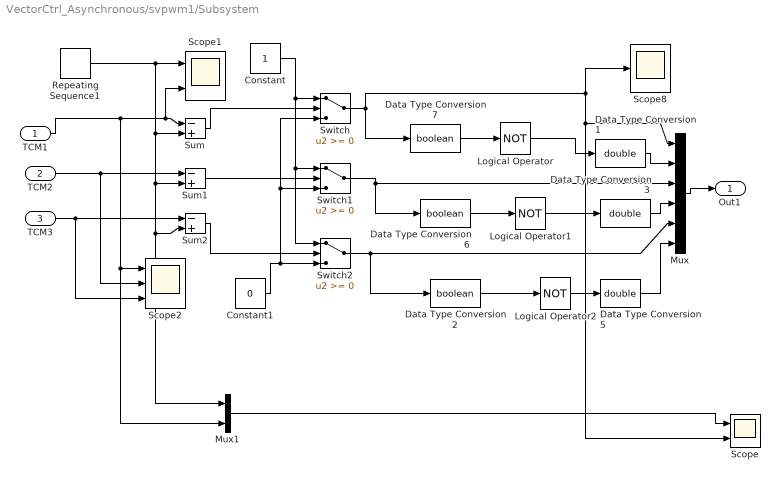
== system VectorCtrl_Asynchronous/svpwm1/Subsystem ==
  TCM1 : Inport
  TCM2 : Inport  Port=2
  TCM3 : Inport  Port=3
  Constant : Constant
  Constant1 : Constant  Value=0
  Data Type Conversion1 : DataTypeConversion  OutDataTypeStr=double  SaturateOnIntegerOverflow=on  RndMeth=Zero
  Data Type Conversion2 : DataTypeConversion  OutDataTypeStr=boolean  SaturateOnIntegerOverflow=on  RndMeth=Zero
  Data Type Conversion3 : DataTypeConversion  OutDataTypeStr=double  SaturateOnIntegerOverflow=on  RndMeth=Zero
  Data Type Conversion5 : DataTypeConversion  OutDataTypeStr=double  SaturateOnIntegerOverflow=on  RndMeth=Zero
  Data Type Conversion6 : DataTypeConversion  OutDataTypeStr=boolean  SaturateOnIntegerOverflow=on  RndMeth=Zero
  Data Type Conversion7 : DataTypeConversion  OutDataTypeStr=boolean  SaturateOnIntegerOverflow=on  RndMeth=Zero
  Logical Operator : Logic  Operator=NOT  AllPortsSameDT=off
  Logical Operator1 : Logic  Operator=NOT  AllPortsSameDT=off
  Logical Operator2 : Logic  Operator=NOT  AllPortsSameDT=off
  Mux : Mux  Inputs=6
  Mux1 : Mux  Inputs=2
  Repeating Sequence1 : simulink/Sources/Repeating Sequence  rep_seq_t=[0 1/10000 1/5000]  rep_seq_y=[0 1/10000 0]
  Scope : Scope  NumInputPorts=2
      settings: YMin=-5~-5  YMax=5~5  SaveName=ScopeData20
  Scope1 : Scope  NumInputPorts=2
      settings: TimeRange=0.028  YMin=0~2.45e-005  YMax=8.5e-005~2.64e-005  SaveName=ScopeData15
  Scope2 : Scope  NumInputPorts=3
      settings: TimeRange=1  YMin=2.25e-005~2.25e-005~2.25e-05  YMax=6e-005~6e-005~6e-05  SaveName=ScopeData19
  Scope8 : Scope
      settings: TimeRange=0.07000000000000001  YMin=0  YMax=2  SaveName=ScopeData13
  Sum : Sum  Inputs=-+  SaturateOnIntegerOverflow=on
  Sum1 : Sum  Inputs=-+  SaturateOnIntegerOverflow=on
  Sum2 : Sum  Inputs=-+  SaturateOnIntegerOverflow=on
  Switch : Switch  SaturateOnIntegerOverflow=on
  Switch1 : Switch  SaturateOnIntegerOverflow=on
  Switch2 : Switch  SaturateOnIntegerOverflow=on
  Out1 : Outport
  wires:
  Constant/1 -> Switch/1, Switch1/1, Switch2/1
  Constant1/1 -> Switch2/3, Switch/3, Switch1/3
  Repeating Sequence1/1 -> Scope1/1, Sum/2, Sum1/2, Sum2/2, Mux1/1
  TCM1/1 -> Sum/1, Scope1/2, Scope2/1, Mux1/2
  TCM2/1 -> Sum1/1, Scope2/2
  TCM3/1 -> Sum2/1, Scope2/3
  Sum/1 -> Switch/2
  Sum1/1 -> Switch1/2
  Sum2/1 -> Switch2/2
  Mux/1 -> Out1/1
  Switch/1 -> Scope8/1, Mux/1, Scope/2, Data Type Conversion7/1
  Switch1/1 -> Mux/3, Data Type Conversion6/1
  Switch2/1 -> Data Type Conversion2/1, Mux/5
  Logical Operator2/1 -> Data Type Conversion5/1
  Logical Operator1/1 -> Data Type Conversion3/1
  Logical Operator/1 -> Data Type Conversion1/1
  Data Type Conversion1/1 -> Mux/2
  Data Type Conversion3/1 -> Mux/4
  Data Type Conversion5/1 -> Mux/6
  Data Type Conversion7/1 -> Logical Operator/1
  Data Type Conversion6/1 -> Logical Operator1/1
  Data Type Conversion2/1 -> Logical Operator2/1
  Mux1/1 -> Scope/1

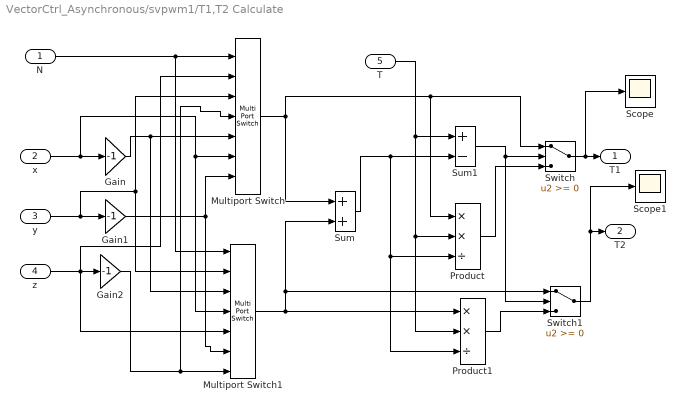
== system VectorCtrl_Asynchronous/svpwm1/T1,T2 Calculate ==
  N : Inport
  x : Inport  Port=2
  y : Inport  Port=3
  z : Inport  Port=4
  T : Inport  Port=5
  Gain : Gain  Gain=-1  SaturateOnIntegerOverflow=on  OutDataTypeStr=Inherit: Same as input  ParamDataTypeStr=Inherit: Same as input
  Gain1 : Gain  Gain=-1  SaturateOnIntegerOverflow=on  OutDataTypeStr=Inherit: Same as input  ParamDataTypeStr=Inherit: Same as input
  Gain2 : Gain  Gain=-1  SaturateOnIntegerOverflow=on  OutDataTypeStr=Inherit: Same as input  ParamDataTypeStr=Inherit: Same as input
  Multiport Switch : MultiPortSwitch  Inputs=6  zeroidx=off  SaturateOnIntegerOverflow=on
  Multiport Switch1 : MultiPortSwitch  Inputs=6  zeroidx=off  SaturateOnIntegerOverflow=on
  Product : Product  Inputs=**/  SaturateOnIntegerOverflow=on  OutDataTypeStr=Inherit: Same as first input
  Product1 : Product  Inputs=**/  SaturateOnIntegerOverflow=on  OutDataTypeStr=Inherit: Same as first input
  Scope : Scope
      settings: YMin=3.5e-005  YMax=6.25e-005  SaveName=ScopeData16
  Scope1 : Scope
      settings: YMin=1.3e-007  YMax=2e-007  SaveName=ScopeData17
  Sum : Sum  SaturateOnIntegerOverflow=on
  Sum1 : Sum  Inputs=+-  SaturateOnIntegerOverflow=on
  Switch : Switch  SaturateOnIntegerOverflow=on
  Switch1 : Switch  SaturateOnIntegerOverflow=on
  T1 : Outport
  T2 : Outport  Port=2
  wires:
  N/1 -> Multiport Switch/1, Multiport Switch1/1
  x/1 -> Gain/1, Multiport Switch/6, Multiport Switch1/4
  y/1 -> Gain1/1, Multiport Switch/3, Multiport Switch1/2
  z/1 -> Gain2/1, Multiport Switch1/5, Multiport Switch/2
  Gain/1 -> Multiport Switch/5, Multiport Switch1/3
  Gain1/1 -> Multiport Switch1/6, Multiport Switch/7
  Gain2/1 -> Multiport Switch1/7, Multiport Switch/4
  Multiport Switch/1 -> Sum/1, Switch/1, Product/1
  Multiport Switch1/1 -> Product1/1, Sum/2, Switch1/1
  Switch1/1 -> T2/1, Scope1/1
  Switch/1 -> T1/1, Scope/1
  T/1 -> Sum1/1, Product1/2, Product/2
  Sum/1 -> Sum1/2, Product1/3, Product/3
  Sum1/1 -> Switch/2, Switch1/2
  Product/1 -> Switch/3
  Product1/1 -> Switch1/3

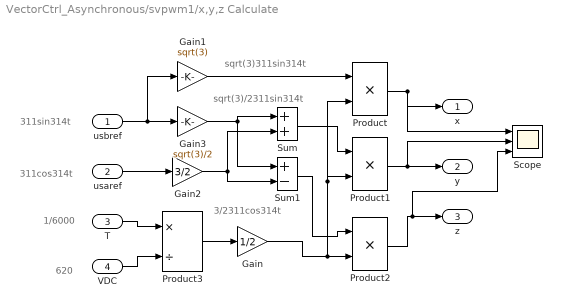
== system VectorCtrl_Asynchronous/svpwm1/x,y,z Calculate ==
  note: 311sin314t
  note: 311cos314t
  note: 1/6000
  note: 620
  note: sqrt(3)311sin314t
  note: sqrt(3)/2311sin314t
  note: 3/2311cos314t
  usbref : Inport
  usaref : Inport  Port=2
  T : Inport  Port=3
  VDC : Inport  Port=4
  Gain : Gain  Gain=1/2  SaturateOnIntegerOverflow=on  OutDataTypeStr=Inherit: Same as input  ParamDataTypeStr=Inherit: Same as input
  Gain1 : Gain  Gain=sqrt(3)  SaturateOnIntegerOverflow=on  OutDataTypeStr=Inherit: Same as input  ParamDataTypeStr=Inherit: Same as input
  Gain2 : Gain  Gain=3/2  SaturateOnIntegerOverflow=on  OutDataTypeStr=Inherit: Same as input  ParamDataTypeStr=Inherit: Same as input
  Gain3 : Gain  Gain=sqrt(3)/2  SaturateOnIntegerOverflow=on  OutDataTypeStr=Inherit: Same as input  ParamDataTypeStr=Inherit: Same as input
  Product : Product  SaturateOnIntegerOverflow=on  OutDataTypeStr=Inherit: Same as first input
  Product1 : Product  SaturateOnIntegerOverflow=on  OutDataTypeStr=Inherit: Same as first input
  Product2 : Product  SaturateOnIntegerOverflow=on  OutDataTypeStr=Inherit: Same as first input
  Product3 : Product  Inputs=*/  SaturateOnIntegerOverflow=on  OutDataTypeStr=Inherit: Same as first input
  Scope : Scope  NumInputPorts=3
      settings: YMin=-8e-005~-8e-005~-8e-005  YMax=8e-005~8e-005~8e-005  SaveName=ScopeData18
  Sum : Sum  SaturateOnIntegerOverflow=on
  Sum1 : Sum  Inputs=+-  SaturateOnIntegerOverflow=on
  x : Outport
  y : Outport  Port=2
  z : Outport  Port=3
  wires:
  T/1 -> Product3/1
  VDC/1 -> Product3/2
  usaref/1 -> Gain2/1
  usbref/1 -> Gain3/1, Gain1/1
  Gain1/1 -> Product/1
  Gain/1 -> Product2/2, Product1/2, Product/2
  Gain3/1 -> Sum/1, Sum1/1
  Gain2/1 -> Sum1/2, Sum/2
  Sum/1 -> Product1/1
  Sum1/1 -> Product2/1
  Product/1 -> x/1, Scope/1
  Product1/1 -> y/1, Scope/2
  Product2/1 -> z/1, Scope/3
  Product3/1 -> Gain/1

== system VectorCtrl_Asynchronous/Controller/Flux Observer/2s/2r1 ==
  αβ : Inport
  sin_cos : Inport  Port=2
  Demux : Demux  Outputs=2
  Demux1 : Demux  Outputs=2
  MATLAB Function : MATLAB Function  TreatAsAtomicUnit=on
  Mux : Mux  Inputs=2
  dq : Outport
  wires:
  Demux1/1 -> MATLAB Function/1(Valpha)
  Demux1/2 -> MATLAB Function/2(Vbeta)
  Mux/1 -> dq/1
  MATLAB Function/2(Vq) -> Mux/2
  Demux/2 -> MATLAB Function/4(coswt)
  Demux/1 -> MATLAB Function/3(sinwt)
  sin_cos/1 -> Demux/1
  αβ/1 -> Demux1/1
  MATLAB Function/1(Vd) -> Mux/1

== system VectorCtrl_Asynchronous/Controller/Flux Observer/Subsystem1 ==
  phi : Inport
  Mux : Mux  Inputs=2
  Trigonometric Function : Trigonometry
  Trigonometric Function1 : Trigonometry  Operator=cos
  sin_cosphi : Outport
  wires:
  phi/1 -> Trigonometric Function/1, Trigonometric Function1/1
  Trigonometric Function/1 -> Mux/1
  Trigonometric Function1/1 -> Mux/2
  Mux/1 -> sin_cosphi/1

== matlab function f_cal/Ramp Function ==
  data: ValueInput input double; ValueAfterRamp output double; AccTime input double; DecTime input double; ValueBase input double; Tsample input double; ValueCurrent input double
function ValueAfterRamp = fcn(ValueInput,AccTime,DecTime,ValueBase, Tsample, ValueCurrent)
%#codegen
%syms ValueCurrent;
%persistent ValueCurrent;
StepAcc = ValueBase*Tsample/AccTime;
StepDec = ValueBase*Tsample/DecTime;
if ValueInput > ValueCurrent;
    if (ValueInput - ValueCurrent)<StepAcc;
        ValueAfterRamp = ValueInput;
    else 
        ValueAfterRamp = ValueCurrent + StepAcc;
    end
elseif ValueInput < ValueCurrent;
    if (ValueCurrent - ValueInput)<StepDec;
        ValueAfterRamp = ValueInput;
    else 
        ValueAfterRamp = ValueCurrent - StepDec;
    end
else 
    ValueAfterRamp = ValueInput;
end
%ValueCurrent = ValueAfterRamp;
%ValueAfterRamp = ValueInput;

== matlab function f_cal/ramp/MATLAB Function ==
  data: ValueInput input double; ValueAfterRamp output double; AccTime input double; DecTime input double; ValueBase input double; Tsample input double; ValueCurrent input double
function ValueAfterRamp = fcn(ValueInput,AccTime,DecTime,ValueBase, Tsample, ValueCurrent)
%#codegen
%syms ValueCurrent;
%persistent ValueCurrent;
StepAcc = ValueBase*Tsample/AccTime;
StepDec = ValueBase*Tsample/DecTime;
if ValueInput > ValueCurrent;
    if (ValueInput - ValueCurrent)<StepAcc;
        ValueAfterRamp = ValueInput;
    else 
        ValueAfterRamp = ValueCurrent + StepAcc;
    end
elseif ValueInput < ValueCurrent;
    if (ValueCurrent - ValueInput)<StepDec;
        ValueAfterRamp = ValueInput;
    else 
        ValueAfterRamp = ValueCurrent - StepDec;
    end
else 
    ValueAfterRamp = ValueInput;
end
%ValueCurrent = ValueAfterRamp;
%ValueAfterRamp = ValueInput;

== matlab function Controller/3s//2s/MATLAB Function ==
  data: Va input double; Valpha output double; Vb input double; Vc input double; Vbeta output double
function [Valpha, Vbeta] = Park(Va, Vb, Vc)
%#codegen
Valpha = sqrt(2/3)*(Va - Vb/2 -Vc/2);
Vbeta  = sqrt(2/3)*(sqrt(3)*Vb/2 - sqrt(3)*Vc/2);

== matlab function Controller/2s//2r/MATLAB Function ==
  data: Valpha input double; Vd output double; Vbeta input double; Vq output double; sinwt input double; coswt input double
function [Vd, Vq] = fcn(Valpha, Vbeta, sinwt, coswt)
%#codegen

Vd =  Valpha*coswt + Vbeta*sinwt;
Vq = -Valpha*sinwt + Vbeta*coswt;

== matlab function Controller/2s//3s/MATLAB Function ==
  data: Va output double; Valpha input double; Vb output double; Vc output double; Vbeta input double
function [Va, Vb, Vc] = Park(Valpha, Vbeta)
%#codegen
Va = sqrt(2/3)*Valpha;
Vb = -Valpha/sqrt(6) + Vbeta/sqrt(2);
Vc = -Valpha/sqrt(6) - Vbeta/sqrt(2);

== matlab function Controller/2r//2s/MATLAB Function ==
  data: Valpha output double; Vd input double; Vbeta output double; Vq input double; sinwt input double; coswt input double
function [Valpha, Vbeta] = fcn(Vd, Vq, sinwt, coswt)
%#codegen

Valpha = Vd*coswt - Vq*sinwt;
Vbeta  = Vd*sinwt + Vq*coswt;

== matlab function Controller/3s//2s1/MATLAB Function ==
  data: Va input double; Valpha output double; Vb input double; Vc input double; Vbeta output double
function [Valpha, Vbeta] = Park(Va, Vb, Vc)
%#codegen
Valpha = sqrt(2/3)*(Va - Vb/2 -Vc/2);
Vbeta  = sqrt(2/3)*(sqrt(3)*Vb/2 - sqrt(3)*Vc/2);

== matlab function Controller/3s//2s2/MATLAB Function ==
  data: Va input double; Valpha output double; Vb input double; Vc input double; Vbeta output double
function [Valpha, Vbeta] = Park(Va, Vb, Vc)
%#codegen
Valpha = sqrt(2/3)*(Va - Vb/2 -Vc/2);
Vbeta  = sqrt(2/3)*(sqrt(3)*Vb/2 - sqrt(3)*Vc/2);

== matlab function Controller/Flux Observer/2s//2r1/MATLAB Function ==
  data: Valpha input double; Vd output double; Vbeta input double; Vq output double; sinwt input double; coswt input double
function [Vd, Vq] = fcn(Valpha, Vbeta, sinwt, coswt)
%#codegen

Vd =  Valpha*coswt + Vbeta*sinwt;
Vq = -Valpha*sinwt + Vbeta*coswt;

== matlab function Line2Phase ==
  data: ValphaL input double; Valpha output double; VbetaL input double; Vbeta output double
function [Valpha, Vbeta] = fcn(ValphaL, VbetaL)
%#将线电压矢量转换成相电压矢量
sin30 = sin(pi/6);
cos30 = cos(pi/6);
Valpha = ( ValphaL*cos30 + VbetaL*sin30)/sqrt(3);
Vbeta  = (-ValphaL*sin30 + VbetaL*cos30)/sqrt(3);

== matlab function Controller/Line2Phase ==
  data: ValphaL input double; Valpha output double; VbetaL input double; Vbeta output double
function [Valpha, Vbeta] = fcn(ValphaL, VbetaL)
%#将线电压矢量转换成相电压矢量
sin30 = sin(pi/6);
cos30 = cos(pi/6);
Valpha = ( ValphaL*cos30 + VbetaL*sin30)/sqrt(3);
Vbeta  = (-ValphaL*sin30 + VbetaL*cos30)/sqrt(3);

== matlab function 2r//2s/MATLAB Function ==
  data: Valpha output double; Vd input double; Vbeta output double; Vq input double; sinwt input double; coswt input double
function [Valpha, Vbeta] = fcn(Vd, Vq, sinwt, coswt)
%#codegen

Valpha = Vd*coswt - Vq*sinwt;
Vbeta  = Vd*sinwt + Vq*coswt;

== matlab function 2s//3s/MATLAB Function ==
  data: Va output double; Valpha input double; Vb output double; Vc output double; Vbeta input double
function [Va, Vb, Vc] = Park(Valpha, Vbeta)
%#codegen
Va = sqrt(2/3)*Valpha;
Vb = -Valpha/sqrt(6) + Vbeta/sqrt(2);
Vc = -Valpha/sqrt(6) - Vbeta/sqrt(2);

== matlab function Controller/Flux Observer/Calc Mod and Angle ==
  data: Valpha input double; Mod output double; Vbeta input double; Angle output double
function [Mod, Angle] = fcn(Valpha, Vbeta)
%Calc Vector Modulus and Angle through alpha and beta value
Mod = sqrt(Valpha*Valpha + Vbeta*Vbeta);
if (Valpha>0)&&(Vbeta>0)
    %第一象限
    Angle = atan(Vbeta/Valpha);
elseif (Valpha>0)&&(Vbeta<0)
    %第四象限
    Angle = atan(Vbeta/Valpha) + 2*pi;
elseif (Valpha<0)&&(Vbeta>0)
    %第二象限
    Angle = atan(Vbeta/Valpha) + pi;
else 
    %第三象限
    Angle = atan(Vbeta/Valpha) + pi;
end

== matlab function Controller/Flux Observer/w Hysteresis ==
  data: u input double; y output double; ubase input double; ybak input double
function y = fcn(u, ubase, ybak)
%#codegen
Threshold = 0.15*ubase;
Hysteresis = 0.05*ubase;
if u>(Threshold+Hysteresis)
    y=1;
elseif u<(Threshold-Hysteresis)
    y=0;
else
    y=ybak;
end

== matlab function CBSVM/2r//2s/MATLAB Function ==
  data: Valpha output double; Vd input double; Vbeta output double; Vq input double; sinwt input double; coswt input double
function [Valpha, Vbeta] = fcn(Vd, Vq, sinwt, coswt)
%#codegen

Valpha = Vd*coswt - Vq*sinwt;
Vbeta  = Vd*sinwt + Vq*coswt;

== matlab function Controller/2r//2s1/MATLAB Function ==
  data: Valpha output double; Vd input double; Vbeta output double; Vq input double; sinwt input double; coswt input double
function [Valpha, Vbeta] = fcn(Vd, Vq, sinwt, coswt)
%#codegen

Valpha = Vd*coswt - Vq*sinwt;
Vbeta  = Vd*sinwt + Vq*coswt;

== matlab function Controller/2s//2r1/MATLAB Function ==
  data: Valpha input double; Vd output double; Vbeta input double; Vq output double; sinwt input double; coswt input double
function [Vd, Vq] = fcn(Valpha, Vbeta, sinwt, coswt)
%#codegen

Vd =  Valpha*coswt + Vbeta*sinwt;
Vq = -Valpha*sinwt + Vbeta*coswt;

== matlab function CBSVM/2s//3s/MATLAB Function ==
  data: Va output double; Valpha input double; Vb output double; Vc output double; Vbeta input double
function [Va, Vb, Vc] = Park(Valpha, Vbeta)
%#codegen
Va = sqrt(2/3)*Valpha;
Vb = -Valpha/sqrt(6) + Vbeta/sqrt(2);
Vc = -Valpha/sqrt(6) - Vbeta/sqrt(2);
